simulink model "AOE_1device"  (R2024b)
settings: Solver=ode4  StartTime=0  StopTime=200  FixedStep=0.01  MaxStep=0.01  RelTol=1e-3
values from neighbouring files (symbols this model uses):
  AOE = Constants_1Device(inputs)    [wecSimInputFile.m]
undefined symbols (not defined in the file or in its folder): body, constraint, DiscIntNeverNeededParam, pto
libraries: WECSim_Lib_Body_Elements x2, simulink x1, WECSim_Lib_Constraints x1, WECSim_Lib_Frames x1, WECSim_Lib_PTOs x1
settings Model: Creator=wcwi  LastModifiedBy=Luke
settings SolverCC: ZeroCrossControl=DisableAll  AlgebraicLoopSolver=TrustRegion  PositivePriorityOrder=on  AutoInsertRateTranBlk=on  InsertRTBMode=Never (minimum delay)
settings DataIOCC: SaveFormat=Array  ReturnWorkspaceOutputs=off
settings OptimizationCC: LifeSpan=inf  SimCompilerOptimization=on  AccelVerboseBuild=on
settings DebuggingCC: UnconnectedInputMsg=warning  UnconnectedOutputMsg=warning  UnconnectedLineMsg=warning  SFUnexpectedBacktrackingDiag=warning  SFNoUnconditionalDefaultTransitionDiag=warning  SFExecutionAtInitializationDiag=none  ArithmeticOperatorsInVariantConditions=warning
settings HardwareCC: ProdBitPerSizeT=32  ProdBitPerPtrDiffT=32  ProdWordSize=32  ProdHWDeviceType=Specified
settings ModelReferenceCC: UpdateModelReferenceTargets=Force  PropagateSignalLabelsOutOfModel=off
settings SFSimCC: SimUseLocalCustomCode=off  CustomCodeUndefinedFunction=UseInterfaceOnly
settings RTWCC: RTWUseLocalCustomCode=off  GPUComputeCapability=3.5
settings CodeAppCC: StateflowObjectComments=on
settings GRTTargetCC: TargetLangStandard=C89/C90 (ANSI)
settings ConfigComp: CovMetricSettings=dw  CovSaveCumulativeToWorkspaceVar=on  CovSaveSingleToWorkspaceVar=on  CovExternalEMLEnable=off

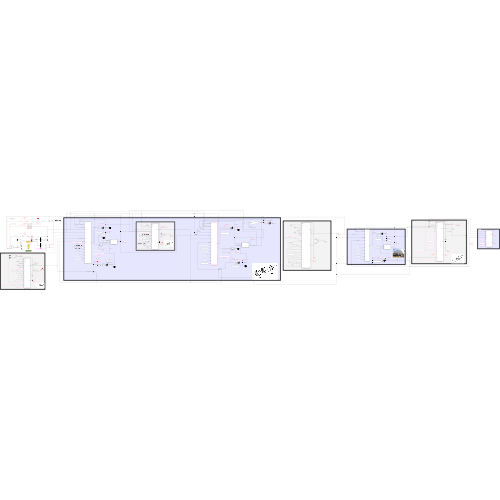
[thumbnail: Simulink's stored preview of the top-level diagram]
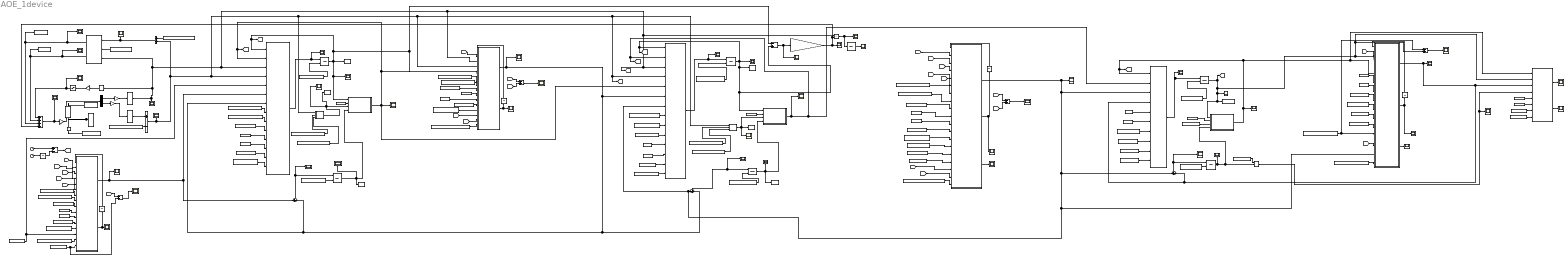
== system AOE_1device ==
  note: Useful Power
  note: Outlet Piston Chamber 1 Valve
  note: Outlet Tank Valve
  note: Inlet Piston valve
  note: Outlet Piston Valve
  " mdot Tank Unit1" : Scope
  " mdot max Tank Unit1" : Scope
  Add1 : Sum  Inputs=+-
  Add{2..3,7,9} (4 alike) : Sum  Inputs=-+
  Add4 : Sum  Inputs=+-  RndMeth=Simplest
  Add8 : Sum  Inputs=++++  RndMeth=Simplest
  Air Mass Chamber1 Unit1 : Scope
  Air Mass Chamber2 Unit1 : Scope
  Air Mass change rate Chamber1 Unit1 : Scope
  Air Mass change rate Chamber2 Unit1 : Scope
  Assertion : Assertion  AssertionFailFcn=Ch1C1 mass is zero
  Assertion1 : Assertion  AssertionFailFcn=Ch1C1 pressure is zero
  Assertion2 : Assertion  AssertionFailFcn=Ch2C1 pressure is zero  StopWhenAssertionFail=off
  Assertion3 : Assertion  AssertionFailFcn=Ch2C1 mass is zero
  Assertion4 : Assertion  AssertionFailFcn=Ch1C1 volume is zero
  Assertion5 : Assertion  AssertionFailFcn=Ch2C1 volume is zero
  Atmospheric pressure1 : Constant  Value=AOE.AtmPressure
  Atmospheric pressure2 : Constant  Value=AOE.AtmPressure
  Bus Selector : BusSelector  OutputSignals=velocity,position
  Chamber pressure potential Unit1 : Scope
  Clock : Clock
  Clock1 : Clock
  Constant{1,14,24,37,56} (5 alike) : Constant  Value=AOE.Unit1.Cylinder.HeatConvection
  Constant{3..5,10,22,27,30,35,39,43,61} (11 alike) : Constant  Value=AOE.Rs
  Constant11 : Constant  Value=AOE.Cp
  Constant16 : Constant  Value=AOE.Unit1.Chamber2.InitialPistonPosition
  Constant17 : Constant  Value=AOE.Unit1.Cylinder.Diameter
  Constant18 : Constant  Value=AOE.Unit1.Chamber2.InitialAirMass
  Constant19 : Constant  Value=AOE.Unit1.Chamber1.InitialPressure
  Constant{2,48,50,55,60} (5 alike) : Constant  Value=AOE.Unit1.Tank.Volume
  Constant20 : Constant  Value=AOE.Unit1.Chamber2.InitialPressure
  Constant21 : Constant  Value=AOE.Unit1.OutletTankOrifice.CrossSectionalArea
  Constant{6,23,28,31,40,47,62} (7 alike) : Constant  Value=AOE.gma
  Constant25 : Constant  Value=AOE.Unit1.Tank.InitialAirMass
  Constant{8,26,38,42,52,57,64} (7 alike) : Constant  Value=AOE.WaterTemperature
  Constant{7,29,41,46,49,51,63} (7 alike) : Constant  Value=AOE.Unit1.Cylinder.CrossSectionalArea
  Constant32 : Constant  Value=AOE.Unit1.Tank.HeatConvection
  Constant33 : Constant  Value=AOE.Unit1.Tank.InitialPressure
  Constant34 : Constant  Value=AOE.Unit1.Tank.SurfaceArea
  Constant44 : Constant  Value=AOE.Unit1.Chamber2.InitialPistonPosition
  Constant53 : Constant  Value=AOE.Unit1.Tank.HeatConvection
  Constant54 : Constant  Value=AOE.Unit1.Tank.SurfaceArea
  Constant58 : Constant  Value=AOE.Unit1.Tank.HeatConvection
  Constant59 : Constant  Value=AOE.Unit1.Tank.SurfaceArea
  Constant65 : Constant  Value=AOE.Unit1.InletCylinderOrifice.CrossSectionalArea
  Constant66 : Constant  Value=AOE.Unit1.OutletCylinderOrifice.CrossSectionalArea
  Constant67 : Constant  Value=AOE.Unit1.Chamber1Chamber2Orifice.CrossSectionalArea
  Constant9 : Constant  Value=AOE.Unit1.Chamber1.InitialAirMass
  Coulomb & Viscous Friction Unit1 : simulink/Discontinuities/Coulomb & Viscous Friction  offset=0  gain=AOE.Unit1.Cylinder.CoulombFrictionGain
  Cyl D{,1..3} (4 alike) : Constant  Value=AOE.Unit1.Cylinder.Diameter
  Density : Scope
  Determining Useful Energy : MATLAB Function
      settings: MinAlgLoopOccurrences=on
  Discrete-Time Integrator : DiscreteIntegrator  InitialConditionSource=external  InitialCondition=101.3  SampleTime=-1  LimitOutput=on  LowerSaturationLimit=0  ICPrevOutput=DiscIntNeverNeededParam  ICPrevScaledInput=DiscIntNeverNeededParam
  Discrete-Time Integrator1 : DiscreteIntegrator  InitialConditionSource=external  InitialCondition=101.3  SampleTime=-1  LimitOutput=on  LowerSaturationLimit=0  ICPrevOutput=DiscIntNeverNeededParam  ICPrevScaledInput=DiscIntNeverNeededParam
  Discrete-Time Integrator10 : DiscreteIntegrator  InitialConditionSource=external  InitialCondition=1.2754*(10)*.25*pi*0.5^2  SampleTime=-1  LimitOutput=on  LowerSaturationLimit=0  ICPrevOutput=DiscIntNeverNeededParam  ICPrevScaledInput=DiscIntNeverNeededParam
  Discrete-Time Integrator11 : DiscreteIntegrator  InitialConditionSource=external  InitialCondition=1.2754*(2+.05)*.25*pi*2.14^2  SampleTime=-1  LimitOutput=on  LowerSaturationLimit=0  ICPrevOutput=DiscIntNeverNeededParam  ICPrevScaledInput=DiscIntNeverNeededParam
  Discrete-Time Integrator12 : DiscreteIntegrator  InitialConditionSource=external  InitialCondition=101.3  SampleTime=-1  LimitOutput=on  LowerSaturationLimit=0  ICPrevOutput=DiscIntNeverNeededParam  ICPrevScaledInput=DiscIntNeverNeededParam
  Discrete-Time Integrator2 : DiscreteIntegrator  InitialConditionSource=external  InitialCondition=1.2754*(2+.05)*.25*pi*2.14^2  SampleTime=-1  LimitOutput=on  LowerSaturationLimit=0  ICPrevOutput=DiscIntNeverNeededParam  ICPrevScaledInput=DiscIntNeverNeededParam
  Endstop Forces Unit1 : Subsystem
  Energy : DiscreteIntegrator  SampleTime=-1  LimitOutput=on  ICPrevOutput=DiscIntNeverNeededParam  ICPrevScaledInput=DiscIntNeverNeededParam
  Energy Unit1 : Scope
  Exergy Unit1 : Scope
  Float : WECSim_Lib_Body_Elements/Rigid Body  body=body(1)
  Floating (6DOF) : WECSim_Lib_Constraints/Floating (6DOF)  constraint=constraint(1)
      settings: AttributesFormatString=%<constraint>
  Gain{,2..4} (4 alike) : Gain  Gain=-1
  Gain1 : Gain  Gain=AOE.Unit1.Cylinder.CrossSectionalArea
  Global Reference Frame : WECSim_Lib_Frames/Global Reference Frame  waves=waves  simu=simu
      settings: SourceProductName=WEC-Sim
  Mech_Energy Unit1 : Scope
  Mech_FTO Unit1 : Scope
  Mech_PTO Unit1 : Scope
  PTO Friction Unit1 : Scope
  Pdot Chamber1 Unit1 : Scope
  Pdot Chamber2 Unit1 : Scope
  Pdot Tank Unit1 : Scope
  Pressure Chamber1 Box Unit1 : MATLAB Function
      settings: MinAlgLoopOccurrences=on
  Pressure Chamber1 Unit1 : Scope
  Pressure Chamber2 Box Unit1 : MATLAB Function
  Pressure Chamber2 Unit1 : Scope
  Pressure Difference Chamb. 1 Unit1 : Scope
  Pressure Difference Cyl. Unit1 : Scope
  Pressure Difference Inlet Unit1 : Scope
  Pressure Difference Tank Unit1 : Scope
  Pressure Tank Box Unit1 : MATLAB Function
      settings: MinAlgLoopOccurrences=on
  Pressure Tank Unit1 : Scope
  Product2 : Product
  Product3 : Product  Inputs=/*
  Revised Cylinder Outlet Valve Model : MATLAB Function
      settings: MinAlgLoopOccurrences=on
  Revised Valve Model Chamber1Chamber2 Unit1 : MATLAB Function
      settings: MinAlgLoopOccurrences=on
  Revised Valve Model Inlet Unit1 : MATLAB Function
      settings: MinAlgLoopOccurrences=on
  Revised Valve Tank Outlet : MATLAB Function
      settings: MinAlgLoopOccurrences=on
  Saturation : Saturate  UpperLimit=AOE.Unit1.Cylinder.CoulombFrictionLimit  LowerLimit=-AOE.Unit1.Cylinder.CoulombFrictionLimit
  Selector : Selector  InputPortWidth=6  IndexOptions=Index vector (dialog)  Indices=3  OutputSizes=1
  Selector1 : Selector  InputPortWidth=6  IndexOptions=Index vector (dialog)  Indices=3  OutputSizes=1
  Spar : WECSim_Lib_Body_Elements/Rigid Body  body=body(2)
  Sum : Sum  Inputs=+-
  Sum1 : Sum  Inputs=-+
  Sum2 : Sum  Inputs=-+
  Sum3 : Sum  Inputs=+|-
  Sum6 : Sum
  Tank Air Mass Unit1 : Scope
  Tank Air Mass change rate Unit1 : Scope
  Temp Chamber1 Unit1 : Scope
  Temp Chamber2 Unit1 : Scope
  Temp Tank Unit1 : Scope
  Temperature Chamber1 Box Unit1 : MATLAB Function  TreatAsAtomicUnit=on
  Temperature Chamber2 Box Unit1 : MATLAB Function
      settings: MinAlgLoopOccurrences=on
  Temperature Tank Box Unit1 : MATLAB Function
  To Workspace : ToWorkspace  VariableName=Fh  SampleTime=-1
  To Workspace1 : ToWorkspace  VariableName=Fl  SampleTime=-1
  To Workspace2 : ToWorkspace  VariableName=PT  SampleTime=-1
  Total Reaction Force : Scope
  Translational PTO Actuation Force : WECSim_Lib_PTOs/Translational PTO Actuation Force  pto=pto(1)
      settings: AttributesFormatString=%<pto>
  Unit Delay{,1..4} (5 alike) : UnitDelay  SampleTime=-1  HasFrameUpgradeWarning=on
  Vol Chamber1 Unit1 : Scope
  Vol Chamber2 Unit1 : Scope
  Volume Chamber1 Box Unit1 : MATLAB Function  TreatAsAtomicUnit=on
  Volume Chamber2 Box Unit1 : MATLAB Function  TreatAsAtomicUnit=on
  beta Cylinder Unit1 : Scope
  beta Unit1 : Scope
  cylinder equilibrium offset position{1,3..5} (4 alike) : Constant  Value=AOE.Unit1.Chamber1.InitialPistonPosition
  cylinder equilibrium offset position2 : Constant  Value=AOE.Unit1.Chamber2.InitialPistonPosition
  cylinder equilibrium offset position6 : Constant  Value=AOE.Unit1.Chamber2.InitialPistonPosition
  cylinder initial offset : Constant  Value=AOE.Unit1.Cylinder.InitialOffset
  cylinder total Length : Constant  Value=AOE.Unit1.Cylinder.Length
  joint F stop high Unit1 : Scope
  joint F stop low Unit1 : Scope
  joint position1 : Scope
  mdot Chamber1Chamber2 Unit1 : Scope
  mdot Cylinder Unit1 : Scope
  mdot Inlet Unit1 : Scope
  mdot Max Chamber1Chamber2 Unit1 : Scope
  mdot Max Cylinder Unit1 : Scope
  mdot max Inlet Unit1 : Scope
  override2 : Constant  Value=AOE.Unit1.OutletTankCheckValve.CrackPressure
  piston position Unit1 : Scope
  piston velocity Unit1 : Scope
  tempAmb1 : Constant  Value=AOE.AtmTemperature
  tempAmb2 : Constant  Value=AOE.AtmTemperature
  wires:
  Add8/1 -> Gain4/1, Total Reaction Force/1  "Total Reaction Force"
  Coulomb & Viscous Friction Unit1/1 -> Gain/1
  Saturation/1 -> PTO Friction Unit1/1, Add8/1  "Motion Friction"
  Endstop Forces Unit1/2(F_stop_lo) -> joint F stop low Unit1/1, Add8/2, To Workspace1/1  "Fstop_low"
  cylinder total Length/1 -> Endstop Forces Unit1/2(Total length)
  Sum6/1 -> Endstop Forces Unit1/1(x(t)), joint position1/1  "Piston Position"
  Endstop Forces Unit1/1(F_stop_hi) -> joint F stop high Unit1/1, Add8/3, To Workspace/1  "Fstop_high"
  Gain/1 -> Saturation/1
  Constant44/1 -> Sum6/1
  Add4/1 -> Sum6/2, Volume Chamber1 Box Unit1/1(x), Revised Valve Model Chamber1Chamber2 Unit1/4(x), Pressure Chamber2 Box Unit1/4(x), [x], Volume Chamber2 Box Unit1/1(x), Pressure Chamber1 Box Unit1/4(x), piston position Unit1/1  "x"
  Pressure Chamber1 Box Unit1/1(Pdot) -> Pdot Chamber1 Unit1/1, Discrete-Time Integrator/1  "pdot(t)"
  Sum/1 -> Discrete-Time Integrator11/1, Air Mass change rate Chamber1 Unit1/1  "mdot1-mdot2"
  Discrete-Time Integrator11/1 -> Air Mass Chamber1 Unit1/1, Temperature Chamber1 Box Unit1/4(m), Assertion/1  "chamber1 air mass"
  Discrete-Time Integrator/1 -> Pressure Chamber1 Box Unit1/1(P), [PC1], Revised Valve Model Chamber1Chamber2 Unit1/5(PC1), Sum1/1, Assertion1/1, Pressure Chamber1 Unit1/1, Temperature Chamber1 Box Unit1/1(P)  "Chamber1 Pressure"
  cylinder equilibrium offset position4/1 -> Pressure Chamber1 Box Unit1/8(L)
  Cyl D/1 -> Pressure Chamber1 Box Unit1/10(D)
  Constant9/1 -> Discrete-Time Integrator11/2
  Constant5/1 -> Pressure Chamber1 Box Unit1/11(Rs)
  Constant6/1 -> Pressure Chamber1 Box Unit1/12(gma)
  Constant7/1 -> Pressure Chamber1 Box Unit1/9(A)
  Constant8/1 -> Pressure Chamber1 Box Unit1/13(Tw)
  Constant37/1 -> Pressure Chamber1 Box Unit1/14(h)
  Constant19/1 -> Discrete-Time Integrator/2
  Constant3/1 -> Temperature Chamber1 Box Unit1/2(Rs)
  Revised Valve Model Chamber1Chamber2 Unit1/1(MassFlow) -> mdot Chamber1Chamber2 Unit1/1, Sum2/2, Pressure Chamber1 Box Unit1/7(mdot3), Sum/2, Pressure Chamber2 Box Unit1/6(mdot1)  "mdot(t)"
  Pressure Chamber2 Box Unit1/1(Pdot) -> Pdot Chamber2 Unit1/1, Discrete-Time Integrator12/1  "pdot(t)"
  Volume Chamber2 Box Unit1/1(V) -> Vol Chamber2 Unit1/1, Assertion5/1, Temperature Chamber2 Box Unit1/3(V)  "Chamber2 volume"
  Sum2/1 -> Discrete-Time Integrator2/1, Air Mass change rate Chamber2 Unit1/1
  Discrete-Time Integrator2/1 -> Temperature Chamber2 Box Unit1/4(m), Air Mass Chamber2 Unit1/1, Assertion3/1  "Chamber2 air mass"
  Constant18/1 -> Discrete-Time Integrator2/2
  Temperature Chamber2 Box Unit1/1(T) -> Temp Chamber2 Unit1/1, Pressure Chamber2 Box Unit1/2(T), [TC2], Pressure Tank Box Unit1/2(Tin)  "Chamber2 temperature"
  Constant16/1 -> Pressure Chamber2 Box Unit1/8(L)
  Constant17/1 -> Pressure Chamber2 Box Unit1/10(D)
  Constant20/1 -> Discrete-Time Integrator12/2
  Constant24/1 -> Pressure Chamber2 Box Unit1/14(h)
  Constant27/1 -> Pressure Chamber2 Box Unit1/11(Rs)
  Constant28/1 -> Pressure Chamber2 Box Unit1/12(gma)
  Constant29/1 -> Pressure Chamber2 Box Unit1/9(A)
  Constant26/1 -> Pressure Chamber2 Box Unit1/13(Tw)
  Constant4/1 -> Temperature Chamber2 Box Unit1/2(Rs)
  Temperature Chamber1 Box Unit1/1(T) -> Pressure Chamber2 Box Unit1/5(Tin1), Temp Chamber1 Unit1/1, Pressure Chamber1 Box Unit1/2(T), [TC1], Revised Valve Model Chamber1Chamber2 Unit1/6(TC1)  "chamber1 temp"
  Revised Cylinder Outlet Valve Model/1(MassFlow) -> Revised Valve Tank Outlet/13(mDotIn), Pressure Chamber2 Box Unit1/7(mdot3), Sum2/1, Sum3/1, Pressure Tank Box Unit1/3(mdot1), mdot Cylinder Unit1/1  "Outlet cylinder"
  Gain1/1 -> Add8/4, Product2/2, Mech_FTO Unit1/1  "Pressure Potential Force"
  Sum1/1 -> Chamber pressure potential Unit1/1, Gain1/1
  Product2/1 -> Energy/1, Mech_PTO Unit1/1
  Energy/1 -> Mech_Energy Unit1/1
  Discrete-Time Integrator12/1 -> Pressure Chamber2 Box Unit1/1(P), [PC2], Pressure Chamber2 Unit1/1, Assertion2/1, Temperature Chamber2 Box Unit1/1(P), Sum1/2  "Chamber2 Pressure"
  Volume Chamber1 Box Unit1/1(V) -> Vol Chamber1 Unit1/1, Assertion4/1, Temperature Chamber1 Box Unit1/3(V)  "Chamber1 Volume"
  cylinder equilibrium offset position1/1 -> Volume Chamber1 Box Unit1/3(L)
  Constant46/1 -> Volume Chamber1 Box Unit1/2(A)
  cylinder equilibrium offset position2/1 -> Volume Chamber2 Box Unit1/3(L)
  Constant49/1 -> Volume Chamber2 Box Unit1/2(A)
  Pressure Tank Box Unit1/1(Pdot) -> Pdot Tank Unit1/1, Discrete-Time Integrator1/1
  Sum3/1 -> Tank Air Mass change rate Unit1/1, Discrete-Time Integrator10/1  "mdot1-mdot2"
  Discrete-Time Integrator10/1 -> Product3/2, Temperature Tank Box Unit1/4(m), Tank Air Mass Unit1/1  "Tank air mas"
  Constant25/1 -> Discrete-Time Integrator10/2
  Constant30/1 -> Pressure Tank Box Unit1/5(Rs)
  Constant31/1 -> Pressure Tank Box Unit1/6(gma)
  Constant32/1 -> Pressure Tank Box Unit1/7(h)
  Constant33/1 -> Discrete-Time Integrator1/2
  Constant34/1 -> Pressure Tank Box Unit1/8(a)
  Constant38/1 -> Pressure Tank Box Unit1/10(Tw)
  Constant50/1 -> Pressure Tank Box Unit1/9(V)
  Constant35/1 -> Temperature Tank Box Unit1/2(Rs)
  Constant48/1 -> Temperature Tank Box Unit1/3(V)
  Temperature Tank Box Unit1/1(T) -> Temp Tank Unit1/1, Revised Valve Tank Outlet/4(TT), Determining Useful Energy/1(T), Pressure Tank Box Unit1/1(T), [TT]  "Unit1 Tank temp"
  Discrete-Time Integrator1/1 -> [PT], To Workspace2/1, Temperature Tank Box Unit1/1(P), Pressure Tank Unit1/1, Revised Valve Tank Outlet/3(PT), Determining Useful Energy/2(P), Add3/2  "Tank pressure"
  override2/1 -> Add3/1, Revised Valve Tank Outlet/11(Pcrack)
  Constant14/1 -> Revised Cylinder Outlet Valve Model/13(hC)
  Constant52/1 -> Revised Cylinder Outlet Valve Model/12(Tw)
  Constant47/1 -> Revised Cylinder Outlet Valve Model/11(gma)
  Constant43/1 -> Revised Cylinder Outlet Valve Model/10(Rs)
  Cyl D1/1 -> Revised Cylinder Outlet Valve Model/9(DC)
  Constant51/1 -> Revised Cylinder Outlet Valve Model/8(AC)
  cylinder equilibrium offset position6/1 -> Revised Cylinder Outlet Valve Model/7(LC)
  Clock1/1 -> Unit Delay1/1
  Unit Delay1/1 -> Add1/2
  Clock/1 -> Add1/1
  Add1/1 -> [TimeStep]
  [TimeStep] -> Revised Cylinder Outlet Valve Model/2(TimeStep)
  Constant53/1 -> Revised Cylinder Outlet Valve Model/14(hT)
  Constant54/1 -> Revised Cylinder Outlet Valve Model/15(aT)
  Constant55/1 -> Revised Cylinder Outlet Valve Model/16(VT)
  [PC2] -> Revised Cylinder Outlet Valve Model/3(PC)
  [TC2] -> Revised Cylinder Outlet Valve Model/4(TC)
  [xDot] -> Revised Cylinder Outlet Valve Model/5(xdot)
  [x] -> Revised Cylinder Outlet Valve Model/6(x)
  [TT] -> Revised Cylinder Outlet Valve Model/18(TT)
  [PT] -> Add2/1
  [PC2] -> Add2/2
  Add2/1 -> Pressure Difference Cyl. Unit1/1
  [PT] -> Revised Cylinder Outlet Valve Model/17(PT)
  [TimeStep] -> Revised Valve Tank Outlet/2(TimeStep)
  Constant57/1 -> Revised Valve Tank Outlet/7(Tw)
  Constant23/1 -> Revised Valve Tank Outlet/6(gma)
  Constant22/1 -> Revised Valve Tank Outlet/5(Rs)
  Constant58/1 -> Revised Valve Tank Outlet/8(hT)
  Constant59/1 -> Revised Valve Tank Outlet/10(aT)
  Constant60/1 -> Revised Valve Tank Outlet/9(VT)
  [TC2] -> Revised Valve Tank Outlet/12(TC)
  Revised Valve Tank Outlet/1(MassFlow) -> Sum3/2, Pressure Tank Box Unit1/4(mdot2), Determining Useful Energy/3(mDot), " mdot Tank Unit1"/1  "Unit1 Outlet tank mdot"
  Constant21/1 -> Revised Valve Tank Outlet/14(A)
  Revised Valve Tank Outlet/2(mdotMax) -> Unit Delay/1, " mdot max Tank Unit1"/1
  Revised Valve Model Inlet Unit1/1(MassFlow) -> Sum/1, Pressure Chamber1 Box Unit1/6(mdot1), mdot Inlet Unit1/1  "Inlet Cylinder MassFlow to Cyl"
  Constant56/1 -> Revised Valve Model Inlet Unit1/13(hC)
  Constant64/1 -> Revised Valve Model Inlet Unit1/12(Tw)
  Constant62/1 -> Revised Valve Model Inlet Unit1/11(gma)
  Constant61/1 -> Revised Valve Model Inlet Unit1/10(Rs)
  Cyl D2/1 -> Revised Valve Model Inlet Unit1/9(DC)
  Constant63/1 -> Revised Valve Model Inlet Unit1/8(AC)
  cylinder equilibrium offset position5/1 -> Revised Valve Model Inlet Unit1/7(LC)
  [TimeStep] -> Revised Valve Model Inlet Unit1/2(TimeStep)
  [PC1] -> Revised Valve Model Inlet Unit1/3(PC1)
  [TC1] -> Revised Valve Model Inlet Unit1/4(TC1)
  [xDot] -> Revised Valve Model Inlet Unit1/5(xdot)
  [x] -> Revised Valve Model Inlet Unit1/6(x)
  Constant65/1 -> Revised Valve Model Inlet Unit1/15(A)
  tempAmb1/1 -> Revised Valve Model Inlet Unit1/14(Tamb), Pressure Chamber1 Box Unit1/5(Tin1)
  Atmospheric pressure1/1 -> Revised Valve Model Inlet Unit1/16(Pamb), Add9/2
  Revised Valve Model Inlet Unit1/2(mdotMax) -> mdot max Inlet Unit1/1, Unit Delay4/1
  Constant66/1 -> Revised Cylinder Outlet Valve Model/19(A)
  cylinder equilibrium offset position3/1 -> Revised Valve Model Chamber1Chamber2 Unit1/7(LC)
  Cyl D3/1 -> Revised Valve Model Chamber1Chamber2 Unit1/9(DC)
  Constant39/1 -> Revised Valve Model Chamber1Chamber2 Unit1/10(Rs)
  Constant40/1 -> Revised Valve Model Chamber1Chamber2 Unit1/11(gma)
  Constant42/1 -> Revised Valve Model Chamber1Chamber2 Unit1/12(Tw)
  Constant1/1 -> Revised Valve Model Chamber1Chamber2 Unit1/13(hC)
  Constant41/1 -> Revised Valve Model Chamber1Chamber2 Unit1/8(AC)
  [TimeStep] -> Revised Valve Model Chamber1Chamber2 Unit1/2(TimeStep)
  [PC2] -> Revised Valve Model Chamber1Chamber2 Unit1/14(PC2)
  [TC2] -> Revised Valve Model Chamber1Chamber2 Unit1/15(TC2)
  Constant67/1 -> Revised Valve Model Chamber1Chamber2 Unit1/16(A)
  Revised Valve Model Chamber1Chamber2 Unit1/2(mdotMax) -> mdot Max Chamber1Chamber2 Unit1/1, Unit Delay3/1
  Add3/1 -> Pressure Difference Tank Unit1/1
  [PC2] -> Add7/1
  [PC1] -> Add7/2
  Add7/1 -> Pressure Difference Chamb. 1 Unit1/1
  [PC1] -> Add9/1
  Add9/1 -> Pressure Difference Inlet Unit1/1
  Revised Cylinder Outlet Valve Model/2(mdotMax) -> Unit Delay2/1, mdot Max Cylinder Unit1/1
  Constant2/1 -> Product3/1
  Product3/1 -> Determining Useful Energy/4(Density), Density/1
  Constant10/1 -> Determining Useful Energy/6(Rs)
  Atmospheric pressure2/1 -> Determining Useful Energy/8(Pamb)
  tempAmb2/1 -> Determining Useful Energy/7(Tamb)
  Constant11/1 -> Determining Useful Energy/5(Cp)
  Determining Useful Energy/1(Exergy) -> Exergy Unit1/1
  Determining Useful Energy/2(Power) -> Energy Unit1/1
  cylinder initial offset/1 -> Add4/2
  Revised Valve Tank Outlet/3(beta) -> beta Unit1/1
  Revised Cylinder Outlet Valve Model/3(beta) -> beta Cylinder Unit1/1
  Unit Delay/1 -> Revised Valve Tank Outlet/1(mdotMaxOld)
  Unit Delay2/1 -> Revised Cylinder Outlet Valve Model/1(mdotMaxOld)
  Unit Delay3/1 -> Revised Valve Model Chamber1Chamber2 Unit1/1(mdotMaxOld)
  Unit Delay4/1 -> Revised Valve Model Inlet Unit1/1(mdotMaxOld)
  Bus Selector/1 -> Gain3/1  "<velocity>"
  Translational PTO Actuation Force/1 -> Bus Selector/1
  Bus Selector/2 -> Gain2/1  "<position>"
  Selector1/1 -> Add4/1
  Selector/1 -> Endstop Forces Unit1/3(xdot(t)), Revised Valve Model Chamber1Chamber2 Unit1/3(xdot), Pressure Chamber2 Box Unit1/3(xdot), [xDot], Product2/1, Pressure Chamber1 Box Unit1/3(xdot), Coulomb & Viscous Friction Unit1/1, piston velocity Unit1/1
  Gain2/1 -> Selector1/1
  Gain3/1 -> Selector/1
  Gain4/1 -> Translational PTO Actuation Force/1
  connections:
  Spar/RConn1 -- Floating (6DOF)/RConn1 -- Translational PTO Actuation Force/LConn1
  Floating (6DOF)/LConn1 -- Global Reference Frame/RConn1
  Translational PTO Actuation Force/RConn1 -- Float/RConn1

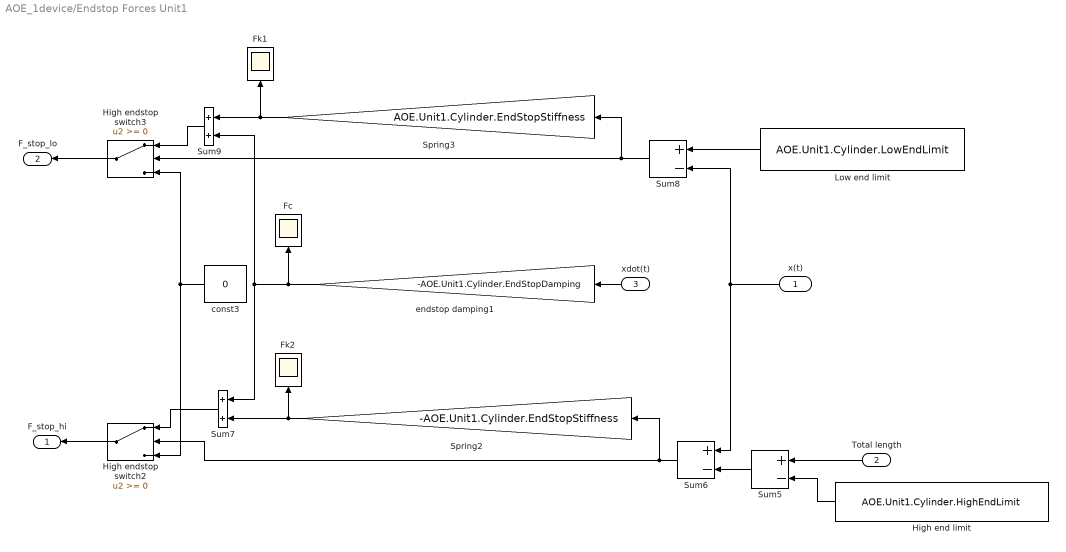
== system AOE_1device/Endstop Forces Unit1 ==
  x(t) : Inport
  Total length : Inport  Port=2
  xdot(t) : Inport  Port=3
  Fc : Scope
  Fk1 : Scope
  Fk2 : Scope
  High end limit : Constant  Value=AOE.Unit1.Cylinder.HighEndLimit
  High endstop switch2 : Switch  SaturateOnIntegerOverflow=off  InputSameDT=off
  High endstop switch3 : Switch  SaturateOnIntegerOverflow=off  InputSameDT=off
  Low end limit : Constant  Value=AOE.Unit1.Cylinder.LowEndLimit
  Spring2 : Gain  Gain=-AOE.Unit1.Cylinder.EndStopStiffness
  Spring3 : Gain  Gain=AOE.Unit1.Cylinder.EndStopStiffness
  Sum5 : Sum  Inputs=+-
  Sum6 : Sum  Inputs=+-
  Sum7 : Sum
  Sum8 : Sum  Inputs=+-
  Sum9 : Sum
  const3 : Constant  Value=0
  endstop damping1 : Gain  Gain=-AOE.Unit1.Cylinder.EndStopDamping
  F_stop_hi : Outport
  F_stop_lo : Outport  Port=2
  wires:
  x(t)/1 -> Sum8/2, Sum6/1
  Total length/1 -> Sum5/1
  High end limit/1 -> Sum5/2
  Sum5/1 -> Sum6/2
  Sum6/1 -> High endstop switch2/2, Spring2/1
  Spring2/1 -> Fk2/1, Sum7/2
  const3/1 -> High endstop switch3/3, High endstop switch2/3
  High endstop switch2/1 -> F_stop_hi/1
  xdot(t)/1 -> endstop damping1/1
  endstop damping1/1 -> Sum9/2, Sum7/1, Fc/1
  Sum7/1 -> High endstop switch2/1
  Low end limit/1 -> Sum8/1
  Sum8/1 -> High endstop switch3/2, Spring3/1
  Spring3/1 -> Fk1/1, Sum9/1
  Sum9/1 -> High endstop switch3/1
  High endstop switch3/1 -> F_stop_lo/1

== matlab function AOE_1device/Temperature Tank Box Unit1 ==
  data: P input; T output; Rs input; V input; m input
function T = fcn(P,Rs,V,m)

T = P*V/(m*Rs);

== matlab function AOE_1device/Volume Chamber1 Box Unit1 ==
  data: x input; A input; V output; L input
function V = fcn(x,A,L)
V = A*(-x +L);

== matlab function AOE_1device/Volume Chamber2 Box Unit1 ==
  data: x input; A input; V output; L input
function V = fcn(x,A,L)

V = A*(x +L);

== matlab function AOE_1device/Revised Cylinder Outlet Valve Model ==
  data: mdotMaxOld input; TimeStep input; PC input; TC input; xdot input; x input; LC input; AC input; DC input; Rs input; gma input; Tw input; hC input; MassFlow output; hT input; aT input; VT input; PT input; TT input; A input; mdotMax output; beta output
function [MassFlow, mdotMax, beta]   = fcn(mdotMaxOld, TimeStep, PC, TC,xdot ,x, LC,AC, DC,Rs,gma,Tw,hC, hT, aT, VT, PT, TT, A)

if PC >= PT
    beta = PT/PC;
    
    if beta > 0.999
        beta = 0.999;
    end
    
    if beta > 0.5283
        mdotMax = A*PC*sqrt(abs((2*gma/((gma-1)*Rs*TC))*((beta)^(2/gma) - (beta)^((gma+1)/gma)))); %subsonic
    else
        mdotMax = 0.0404*PC*A/sqrt(TC); %sonic
    end
    
else
    mdotMax = 0;
    beta = 0;
end

%Calculating Volumes/Areas
VC = AC*(x +LC);
aC = pi*DC*(x +LC) + 2*AC; %heat transfer area

if TimeStep == 0
    MassFlow = 0;
    %MassFlow_Opt = 0;
    %MassFlow_Opt2 = 0;
    PdotC = 0;
    Change = 0;
else
    Change = 0;
    
    
%     %Determining what the tank properties will be in the next time step
%     
%     PT = PT + Pdot*TimeStep;
%     TT = PT*VT/(Tmass*Rs);
%     
%     %Determining what the cylinder properties will be in the next time step
%     PdotC = (-1*gma*PC*(xdot)*AC - (gma-1)*hC*aC*(TC-Tw) - gma*Rs*TC*MassFlowOld)/VC;
%     PC = PC + PdotC*TimeStep;
%     TC = PC*VC/(Cmass*Rs);
    
    %Determining what the pressure needs to be in the following time step
    %P2 = (TimeStep/(VT+VC))*( (PT*VT/TimeStep) + (PC*VC/TimeStep) - gma*PC*(xdot)*AC - (gma-1)*hC*aC*(TC-Tw) -(gma-1)*hT*aT*(TT-Tw) + gma*Rs*TT*mDotT);
    P2 = (TimeStep/(VT+VC))*( (PT*VT/TimeStep) + (PC*VC/TimeStep) - gma*PC*(xdot)*AC - (gma-1)*hC*aC*(TC-Tw) -(gma-1)*hT*aT*(TT-Tw));
    
    MassFlow_Opt = (1/(Rs*TC*gma))*( -(P2 - PC)*VC/TimeStep - gma*PC*(xdot)*AC - (gma-1)*hC*aC*(TC-Tw) );
    %MassFlow_Opt2 = (1/(Rs*TC*gma))*( (P2 - PT)*VT/TimeStep + (gma-1)*hT*aT*(TT-Tw) - gma*Rs*TT*mDotT);
    
    MassFlow = MassFlow_Opt*0.99;
    
    PdotC = (-1*gma*PC*(xdot)*AC - (gma-1)*hC*aC*(TC-Tw) - gma*Rs*TC*MassFlow )/VC;
end

if MassFlow < 0
    MassFlow = 0;
end

if MassFlow > mdotMax
    if mdotMaxOld > mdotMax
        if MassFlow > mdotMaxOld
            MassFlow = mdotMaxOld;
        end
        mdotMax = mdotMaxOld;
    else
        MassFlow = mdotMax;
    end
end

% if Change == 1
%     PdotC = (-1*gma*PC*(xdot)*AC - (gma-1)*hC*aC*(TC-Tw) - gma*Rs*TC*MassFlow )/VC;
% end

PCPredicted = PC + PdotC*TimeStep;

== matlab function AOE_1device/Revised Valve Tank Outlet ==
  data: mdotMaxOld input; TimeStep input; PT input; TT input; Rs input; gma input; Tw input; hT input; VT input; aT input; MassFlow output; Pcrack input; TC input; mDotIn input; A input; mdotMax output; beta output
function [MassFlow, mdotMax, beta]   = fcn(mdotMaxOld, TimeStep, PT, TT ,Rs,gma,Tw,hT, VT, aT, Pcrack, TC, mDotIn, A)

%Determine Maximum Mass Flow Rate

%A is orifice area

if PT >= Pcrack
    beta = Pcrack/PT;
    
    %This prevents instabilities as Beta approaches 1
    if beta > 0.999
        beta = 0.999;
    end
    
    if beta > 0.5283
        mdotMax = A*PT*sqrt(abs((2*gma/((gma-1)*Rs*TT))*((beta)^(2/gma) - (beta)^((gma+1)/gma)))); %subsonic
    else
        mdotMax = 0.0404*PT*A/sqrt(TT); %sonic
    end
    
else
    mdotMax = 0;
    beta = 0;
end

if TimeStep == 0
    MassFlow = 0;
else
    %Determining what the pressure needs to be in the following time step
    P2 = Pcrack;
    
    MassFlow_Opt = (1/(Rs*TT*gma))*( -(P2 - PT)*VT/TimeStep - (gma-1)*hT*aT*(TT-Tw) + gma*Rs*TC*mDotIn);
    
    MassFlow = MassFlow_Opt*0.99;
end

if MassFlow < 0
    MassFlow = 0;
end

if MassFlow > mdotMax
    if mdotMaxOld > mdotMax
        if MassFlow > mdotMaxOld
            MassFlow = mdotMaxOld;
        end
        mdotMax = mdotMaxOld;
    else
        MassFlow = mdotMax;
    end
end
    
end

== matlab function AOE_1device/Revised Valve Model Inlet Unit1 ==
  data: mdotMaxOld input; TimeStep input; PC1 input; TC1 input; xdot input; x input; LC input; AC input; DC input; Rs input; gma input; Tw input; hC input; Tamb input; A input; MassFlow output; Pamb input; mdotMax output
function [MassFlow, mdotMax]   = fcn(mdotMaxOld, TimeStep, PC1, TC1,xdot ,x, LC,AC, DC,Rs,gma,Tw,hC, Tamb, A, Pamb)

if Pamb >= PC1
    beta = PC1/Pamb;
    
    if beta > 0.999
        beta = 0.999;
    end
    
    if beta > 0.5283
        mdotMax = A*Pamb*sqrt(abs((2*gma/((gma-1)*Rs*Tamb))*((beta)^(2/gma) - (beta)^((gma+1)/gma)))); %subsonic
    else
        mdotMax = 0.0404*Pamb*A/sqrt(Tamb); %sonic
    end
    
else
    mdotMax = 0;
end

if TimeStep == 0
    MassFlow = 0;
else
    %Calculating Volumes/Areas
    VC = AC*(-x +LC);
    aC = pi*DC*(-x +LC) + 2*AC; %heat transfer area
    
    %Determining what the pressure needs to be in the following time step
    P2 = Pamb;
    
    MassFlow_Opt = (1/(Rs*Tamb*gma))*( (P2 - PC1)*VC/TimeStep + gma*PC1*(-xdot)*AC + (gma-1)*hC*aC*(TC1-Tw) );
    MassFlow = MassFlow_Opt*0.99;

end

if MassFlow < 0
    MassFlow = 0;
end

if MassFlow > mdotMax
    if mdotMaxOld > mdotMax
        if MassFlow > mdotMaxOld
            MassFlow = mdotMaxOld;
        end
        mdotMax = mdotMaxOld;
    else
        MassFlow = mdotMax;
    end
end

== matlab function AOE_1device/Revised Valve Model Chamber1Chamber2 Unit1 ==
  data: mdotMaxOld input; TimeStep input; xdot input; x input; PC1 input; TC1 input; LC input; AC input; DC input; Rs input; gma input; Tw input; hC input; MassFlow output; PC2 input; TC2 input; A input; mdotMax output
function [MassFlow, mdotMax]   = fcn(mdotMaxOld, TimeStep, xdot ,x,PC1, TC1, LC,AC, DC,Rs,gma,Tw,hC, PC2, TC2, A)

if PC1 >= PC2
    beta = PC2/PC1;
    
    if beta > 0.999
        beta = 0.999;
    end
    
    if beta > 0.5283
        mdotMax = A*PC1*sqrt(abs((2*gma/((gma-1)*Rs*TC1))*((beta)^(2/gma) - (beta)^((gma+1)/gma)))); %subsonic
    else
        mdotMax = 0.0404*PC1*A/sqrt(TC1); %sonic
    end
    
else
    mdotMax = 0;
end

if TimeStep == 0
    MassFlow = 0;
else
    %Calculating Volumes/Areas
    VC1 = AC*(-x +LC);
    aC1 = pi*DC*(-x +LC) + 2*AC; %heat transfer area
    
    VC2 = AC*(x +LC);
    aC2 = pi*DC*(x +LC) + 2*AC; %heat transfer area
    
    %Determining what the pressure needs to be in the following time step
    P2 = (TimeStep/(VC2+VC1))*( (PC2*VC2/TimeStep) + (PC1*VC1/TimeStep) - gma*PC1*(-xdot)*AC - (gma-1)*hC*aC1*(TC1-Tw) - gma*PC2*xdot*AC - (gma-1)*hC*aC2*(TC2-Tw));
    
    MassFlow_Opt = (1/(Rs*TC1*gma))*( -(P2 - PC1)*VC1/TimeStep - gma*PC1*(-xdot)*AC - (gma-1)*hC*aC1*(TC1-Tw) );
    MassFlow = MassFlow_Opt*0.99;

end

if MassFlow < 0
    MassFlow = 0;
end

if MassFlow > mdotMax
    if mdotMaxOld > mdotMax
        if MassFlow > mdotMaxOld
            MassFlow = mdotMaxOld;
        end
        mdotMax = mdotMaxOld;
    else
        MassFlow = mdotMax;
    end
end

== matlab function AOE_1device/Pressure Chamber1 Box Unit1 ==
  data: P input; T input; xdot input; x input; Tin1 input; mdot1 input; mdot3 input; L input; A input; D input; Rs input; gma input; Tw input; h input; Pdot output
function Pdot = fcn(P, T,xdot ,x, Tin1, mdot1,mdot3,L,A, D,Rs,gma,Tw,h)

V = A*(-x +L);
a = pi*D*(-x +L) + 2*A; %heat transfer area

Pdot = (-1*gma*P*(-xdot)*A - (gma-1)*h*a*(T-Tw) + gma*Rs*Tin1*mdot1 - gma*Rs*T*mdot3)/V;

== matlab function AOE_1device/Pressure Tank Box Unit1 ==
  data: T input; Tin input; mdot1 input; mdot2 input; Rs input; gma input; h input; a input; V input; Tw input; Pdot output
function Pdot  = fcn(T, Tin, mdot1,mdot2,Rs,gma,h, a, V,Tw)

Pdot = (-(gma-1)*h*a*(T-Tw) + gma*Rs*Tin*mdot1 - gma*Rs*T*mdot2)/V;

== matlab function AOE_1device/Determining Useful Energy ==
  data: T input; P input; mDot input; Density input; Cp input; Rs input; Tamb input; Pamb input; Exergy output; Power output
function [Exergy, Power]   = fcn(T, P, mDot, Density, Cp, Rs, Tamb, Pamb)
    
%Determining Flow Exergy
Flow_Exergy = Cp*Tamb*( (T/Tamb) - 1 - log(T/Tamb) ) + Rs*Tamb*log(P/Pamb);

Exergy = Flow_Exergy*mDot; %This has the units of Watts

%Determining Energy of Output
Power = mDot*(P - Pamb)/Density;

end

== matlab function AOE_1device/Temperature Chamber1 Box Unit1 ==
  data: P input; T output; Rs input; V input; m input
function T = fcn(P,Rs,V,m)
T = P*V/(m*Rs);

== matlab function AOE_1device/Pressure Chamber2 Box Unit1 ==
  data: P input; T input; xdot input; x input; Tin1 input; mdot1 input; mdot3 input; L input; A input; D input; Pdot output; Rs input; gma input; Tw input; h input
function Pdot = fcn(P, T,xdot ,x, Tin1, mdot1,mdot3,L,A, D,Rs,gma,Tw,h)

V = A * (x +L);
a = pi*D*(x +L) + 2*A; %heat transfer area

Pdot = (-1*gma*P*(xdot)*A - (gma-1)*h*a*(T-Tw) + gma*Rs*Tin1*mdot1 - gma*Rs*T*mdot3)/V;

== matlab function AOE_1device/Temperature Chamber2 Box Unit1 ==
  data: P input; T output; Rs input; V input; m input
function T = fcn(P,Rs,V,m)

T = P*V/(m*Rs);
